simulink model "single_pendulum"  (R2016a)
settings: Solver=ode23  StartTime=0.0  StopTime=tfinal  RelTol=1e-3
values from neighbouring files (symbols this model uses):
  l = 0.7    [runSimulink_single_pendulum.m]
  m = 1.5    [runSimulink_single_pendulum.m]
settings Model: Creator=dqtm  LastModifiedBy=dqtm
settings DataIOCC: LimitDataPoints=on  SaveFormat=Array  SignalLoggingSaveFormat=ModelDataLogs
settings OptimizationCC: ExpressionDepthLimit=2147483647  InitFltsAndDblsToZero=on
settings DebuggingCC: UnderspecifiedInitializationDetection=Classic  MergeDetectMultiDrivingBlocksExec=none  SolverPrmCheckMsg=warning  FcnCallInpInsideContextMsg=UseLocalSettings  StateNameClashWarn=warning
settings HardwareCC: ProdBitPerPointer=32  ProdLargestAtomicFloat=None  ProdIntDivRoundTo=Undefined  ProdEndianess=Unspecified  ProdWordSize=32  ProdHWDeviceType=32-bit Generic
settings ModelReferenceCC: PropagateSignalLabelsOutOfModel=off
settings GRTTargetCC: CombineOutputUpdateFcns=off  GRTInterface=on
settings ConfigComp: CovModelRefEnable=Off

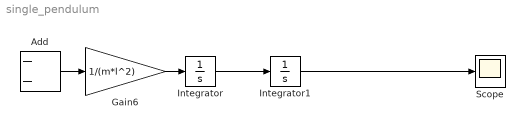
== system single_pendulum ==
  Add : Sum  Inputs=--
  Gain6 : Gain  Gain=1/(m*l^2)
  Integrator : Integrator
  Integrator1 : Integrator
  Scope : Scope
  wires:
  Integrator/1 -> Integrator1/1
  Add/1 -> Gain6/1
  Integrator1/1 -> Scope/1
  Gain6/1 -> Integrator/1
